simulink model "Engines"  (R2017b)
settings: Solver=VariableStepAuto  StartTime=0.0  StopTime=10.0  RelTol=1e-3
settings Model: Creator=zht  LastModifiedBy=zht

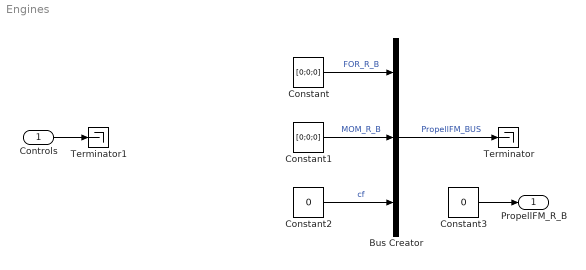
== system Engines ==
  Controls : Inport
  Bus Creator : BusCreator  Inputs=3
  Constant : Constant  Value=[0;0;0]
  Constant1 : Constant  Value=[0;0;0]
  Constant2 : Constant  Value=0
  Constant3 : Constant  Value=0
  Terminator : Terminator
  Terminator1 : Terminator
  PropellFM_R_B : Outport
  wires:
  Bus Creator/1 -> Terminator/1  "PropellFM_BUS"
  Constant2/1 -> Bus Creator/3  "cf"
  Constant1/1 -> Bus Creator/2  "MOM_R_B"
  Constant/1 -> Bus Creator/1  "FOR_R_B"
  Constant3/1 -> PropellFM_R_B/1
  Controls/1 -> Terminator1/1
